simulink model "butterfly"  (R2013a)
settings: Solver=ode45  StartTime=0.0  StopTime=9  RelTol=1e-3
settings Model: Creator=sgowda  LastModifiedBy=sgowda

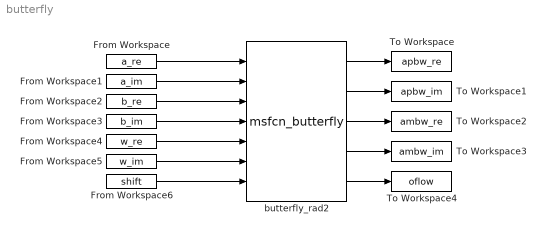
== system butterfly ==
  From Workspace : FromWorkspace  VariableName=a_re  SampleTime=0  Interpolate=off  OutputAfterFinalValue=Setting to zero
  From Workspace1 : FromWorkspace  VariableName=a_im  SampleTime=0  Interpolate=off  OutputAfterFinalValue=Setting to zero
  From Workspace2 : FromWorkspace  VariableName=b_re  SampleTime=0  Interpolate=off  OutputAfterFinalValue=Setting to zero
  From Workspace3 : FromWorkspace  VariableName=b_im  SampleTime=0  Interpolate=off  OutputAfterFinalValue=Setting to zero
  From Workspace4 : FromWorkspace  VariableName=w_re  SampleTime=0  Interpolate=off  OutputAfterFinalValue=Setting to zero
  From Workspace5 : FromWorkspace  VariableName=w_im  SampleTime=0  Interpolate=off  OutputAfterFinalValue=Setting to zero
  From Workspace6 : FromWorkspace  VariableName=shift  SampleTime=0  Interpolate=off  OutputAfterFinalValue=Setting to zero
  To Workspace : ToWorkspace  VariableName=apbw_re  SampleTime=-1
  To Workspace1 : ToWorkspace  VariableName=apbw_im  SampleTime=-1
  To Workspace2 : ToWorkspace  VariableName=ambw_re  SampleTime=-1
  To Workspace3 : ToWorkspace  VariableName=ambw_im  SampleTime=-1
  To Workspace4 : ToWorkspace  VariableName=oflow  SampleTime=-1
  butterfly_rad2 : M-S-Function  FunctionName=msfcn_butterfly
      mask Display:
      | port_label('input', 1, 'a_re');
      | port_label('input', 2, 'a_im');
      | port_label('input', 3, 'b_re');
      | port_label('input', 4, 'b_im');
      | port_label('input', 5, 'w_re');
      | port_label('input', 6, 'w_im');
      | port_label('input', 7, 'shift');
  wires:
  From Workspace/1 -> butterfly_rad2/1
  From Workspace1/1 -> butterfly_rad2/2
  From Workspace2/1 -> butterfly_rad2/3
  From Workspace3/1 -> butterfly_rad2/4
  From Workspace4/1 -> butterfly_rad2/5
  From Workspace5/1 -> butterfly_rad2/6
  From Workspace6/1 -> butterfly_rad2/7
  butterfly_rad2/1 -> To Workspace/1
  butterfly_rad2/2 -> To Workspace1/1
  butterfly_rad2/3 -> To Workspace2/1
  butterfly_rad2/4 -> To Workspace3/1
  butterfly_rad2/5 -> To Workspace4/1
